simulink model "random_gen"  (R2015a)
settings: Solver=ode3  StartTime=0.0  StopTime=20  FixedStep=0.1  RelTol=1e-6
libraries: lib x1
settings Model: SimulationMode=accelerator  CovSFcnEnable=off  Creator=jdeshmukh  LastModifiedBy=alex
settings DataIOCC: LimitDataPoints=off  SignalLoggingSaveFormat=ModelDataLogs  SignalLogging=off  DSMLogging=off
settings DebuggingCC: UnderspecifiedInitializationDetection=Classic  MergeDetectMultiDrivingBlocksExec=none  SolverPrmCheckMsg=warning  MultiTaskDSMMsg=warning  MultiTaskCondExecSysMsg=none  StateNameClashWarn=warning
settings GRTTargetCC: MatFileLogging=off  RTWCAPISignals=on  RTWCAPIParams=on

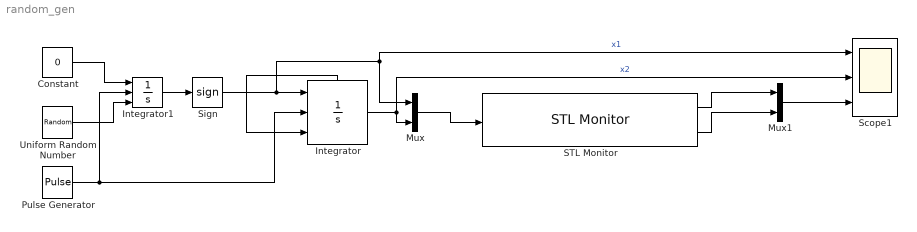
== system random_gen ==
  Constant : Constant  Value=0
  Integrator : Integrator  ExternalReset=rising  InitialConditionSource=external  ShowStatePort=on
  Integrator1 : Integrator  ExternalReset=rising  InitialConditionSource=external
  Mux : Mux  Inputs=2
  Mux1 : Mux  Inputs=2
  Pulse Generator : DiscretePulseGenerator  PulseType=Time based  Period=1  PulseWidth=50
  STL Monitor : lib/STL Monitor  SignalNames='x1,x2'  STLString='x1[t]>0'  MaxRob=100  RefreshRate=0.1  rob_low_lim=inf  rob_up_lim=-inf  rob_diff_lim=-inf
  Scope1 : Scope  NumInputPorts=3
      settings: YMin=0.22~-5~-1.05  YMax=0.44~5~-0.95
  Sign : Signum
  Uniform Random Number : UniformRandomNumber  Minimum=-2  Maximum=2
  wires:
  Integrator/1 -> Mux/2, Scope1/2  "x2"
  Pulse Generator/1 -> Integrator/2, Integrator1/2
  Integrator/State -> Integrator/3
  Sign/1 -> Integrator/1, Mux/1, Scope1/1  "x1"
  Constant/1 -> Integrator1/1
  Uniform Random Number/1 -> Integrator1/3
  Integrator1/1 -> Sign/1
  Mux1/1 -> Scope1/3
  Mux/1 -> STL Monitor/1
  STL Monitor/1 -> Mux1/1
  STL Monitor/2 -> Mux1/2
